simulink model "RectifierAndBuck"  (R2018a)
settings: Solver=VariableStepAuto  StartTime=0.0  StopTime=0.2  MaxStep=1e-5  RelTol=1e-3
libraries: powerlib x21, powerlib_meascontrol x9
settings Model: Creator=oguna  LastModifiedBy=Emre Deniz
settings DebuggingCC: LibraryContextMissingDiagnostic=warning
settings SFSimCC: SimUseLocalCustomCode=on
settings RTWCC: RTWUseLocalCustomCode=on

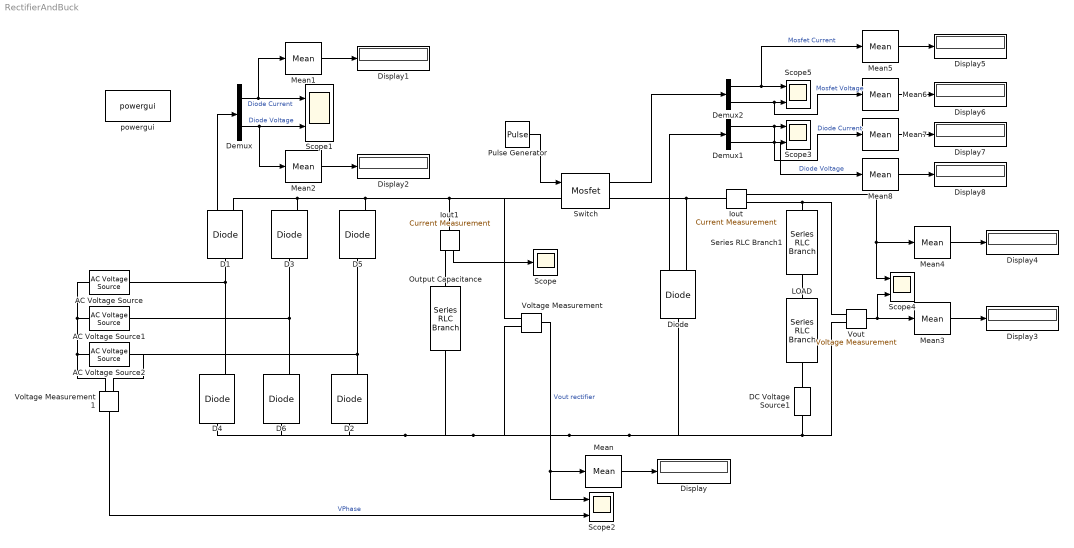
== system RectifierAndBuck ==
  AC Voltage Source : powerlib/Electrical Sources/AC Voltage Source  Amplitude=100*sqrt(2)  Phase=0  Frequency=50  SampleTime=0  Measurements=None  BusType=swing  Pref=10e3  Qref=0  Qmin=-inf  Qmax=+inf
  AC Voltage Source1 : powerlib/Electrical Sources/AC Voltage Source  Amplitude=100*sqrt(2)  Phase=-120  Frequency=50  SampleTime=0  Measurements=None  BusType=swing  Pref=10e3  Qref=0  Qmin=-inf  Qmax=+inf
  AC Voltage Source2 : powerlib/Electrical Sources/AC Voltage Source  Amplitude=100*sqrt(2)  Phase=120  Frequency=50  SampleTime=0  Measurements=None  BusType=swing  Pref=10e3  Qref=0  Qmin=-inf  Qmax=+inf
  D{1..6} (6 alike) : powerlib/Power Electronics/Diode  Ron=0  Lon=0  Vf=0  IC=0  UseSnubber=0  Rs=inf  Cs=0  Measurements=on
  DC Voltage Source1 : powerlib/Electrical Sources/DC Voltage Source  Amplitude=0.1  Measurements=None
  Demux : Demux  Outputs=2
  Demux1 : Demux  Outputs=2
  Demux2 : Demux  Outputs=2
  Diode : powerlib/Power Electronics/Diode  Ron=0  Lon=0  Vf=0  IC=0  UseSnubber=0  Rs=inf  Cs=0  Measurements=on
  Display{,1..8} (9 alike) : Display
  Iout : powerlib/Measurements/Current Measurement  PhasorSimulation=off  OutputType=Complex  PSBequivalent=0
  Iout1 : powerlib/Measurements/Current Measurement  PhasorSimulation=off  OutputType=Complex  PSBequivalent=0
  LOAD : powerlib/Elements/Series RLC Branch  LConnTagsString=__new0  RConnTagsString=__new0  BranchType=R  Resistance=1.07  Inductance=1e-3  SetiL0=off  InitialCurrent=0  Capacitance=1e-6  Setx0=off  InitialVoltage=0  Measurements=None
  Mean{,1..8} (9 alike) : powerlib_meascontrol/Measurements/Mean  Freq=50  Vinit=0  Ts=0
  Output Capacitance : powerlib/Elements/Series RLC Branch  LConnTagsString=__new0  RConnTagsString=__new0  BranchType=RC  Resistance=0.0001  Inductance=1e-3  SetiL0=off  InitialCurrent=0  Capacitance=47e-6  Setx0=off  InitialVoltage=0  Measurements=None
  Pulse Generator : DiscretePulseGenerator  PulseType=Time based  Period=1/1000  PulseWidth=10
  Scope : Scope
  Scope{1..5} (5 alike) : Scope  NumInputPorts=2
  Series RLC Branch1 : powerlib/Elements/Series RLC Branch  LConnTagsString=__new0  RConnTagsString=__new0  BranchType=L  Resistance=1  Inductance=24e-3  SetiL0=off  InitialCurrent=0  Capacitance=1e-6  Setx0=off  InitialVoltage=0  Measurements=None
  Switch : powerlib/Power Electronics/Mosfet  Ron=0.1  Lon=0  Rd=0.01  Vfd=0  IC=0  Rs=1e5  Cs=inf  Measurements=on
  Voltage Measurement : powerlib/Measurements/Voltage Measurement  PhasorSimulation=off  OutputType=Complex  PSBequivalent=0
  Voltage Measurement1 : powerlib/Measurements/Voltage Measurement  PhasorSimulation=off  OutputType=Complex  PSBequivalent=0
  Vout : powerlib/Measurements/Voltage Measurement  PhasorSimulation=off  OutputType=Complex  PSBequivalent=0
  powergui : powerlib/powergui  Priority=1  SimulationMode=Continuous  SampleTime=50e-6  frequency=60  Iterations=50  frequencyindice=50  Pbase=100e6  ErrMax=1e-4  UnitsV=kV  UnitsW=MW  buscounter=0  FunctionMessages=off  echomessages=off  EnableUseOfTLC=off  CurrentSourceSwitches=off  DisableSnubberDevices=off  DisableRonSwitches=off  DisableVfSwitches=off  DisplayEquations=off  SolverType=Tustin/Backward Euler (TBE)  Interpol=off  ExternalGateDelay=off  methode=off  Ts=100  x0status=blocks  SPID=on  SwTol=0  HookPort=off  RestoreLinks=warning  ResistiveCurrentMeasurement=off  Frange=[0:2:500]  Ylog=off  Xlog=on  ShowGrid=off  save=off  variable=ZData  structure=0  ZoomFFT=off  StartTime=0.0  cycles=1  DisplayStyle=1  fundamental=60  FreqAxis=off  MaxFrequency=1000  frequencyindicesteady=1  RmsSteady=1  display=off
  wires:
  Voltage Measurement/1 -> Scope2/1, Mean/1  "Vout rectifier"
  Mean/1 -> Display/1
  D1/1 -> Demux/1
  Demux/2 -> Mean2/1, Scope1/2  "Diode Voltage"
  Demux/1 -> Mean1/1, Scope1/1  "Diode Current"
  Voltage Measurement1/1 -> Scope2/2  "VPhase"
  Diode/1 -> Demux1/1
  Demux2/2 -> Mean6/1, Scope5/2  "Mosfet Voltage"
  Switch/1 -> Demux2/1
  Demux2/1 -> Mean5/1, Scope5/1  "Mosfet Current"
  Demux1/1 -> Mean7/1, Scope3/1  "Diode Current"
  Demux1/2 -> Mean8/1, Scope3/2  "Diode Voltage"
  Pulse Generator/1 -> Switch/1
  Mean1/1 -> Display1/1
  Mean2/1 -> Display2/1
  Vout/1 -> Mean3/1, Scope4/2
  Mean3/1 -> Display3/1
  Mean4/1 -> Display4/1
  Iout/1 -> Mean4/1, Scope4/1
  Mean5/1 -> Display5/1
  Mean6/1 -> Display6/1
  Mean7/1 -> Display7/1
  Mean8/1 -> Display8/1
  Iout1/1 -> Scope/1
  connections:
  AC Voltage Source/LConn1 -- Voltage Measurement1/LConn2 -- AC Voltage Source2/LConn1 -- AC Voltage Source1/LConn1
  D1/LConn1 -- AC Voltage Source/RConn1 -- D4/RConn1
  D3/LConn1 -- AC Voltage Source1/RConn1 -- D6/RConn1
  D5/LConn1 -- Voltage Measurement1/LConn1 -- AC Voltage Source2/RConn1 -- D2/RConn1
  D1/RConn1 -- Iout1/LConn1 -- Voltage Measurement/LConn1 -- Switch/LConn1 -- D5/RConn1 -- D3/RConn1
  Vout/LConn2 -- DC Voltage Source1/LConn1 -- Diode/LConn1 -- Voltage Measurement/LConn2 -- Output Capacitance/RConn1 -- D2/LConn1 -- D4/LConn1 -- D6/LConn1
  Vout/LConn1 -- Series RLC Branch1/LConn1 -- Iout/RConn1
  Switch/RConn1 -- Iout/LConn1 -- Diode/RConn1
  DC Voltage Source1/RConn1 -- LOAD/RConn1
  Series RLC Branch1/RConn1 -- LOAD/LConn1
  Iout1/RConn1 -- Output Capacitance/LConn1
